simulink model "stateflow_test"  (R2020a)
settings: Solver=FixedStepDiscrete  StartTime=0.0  StopTime=inf  FixedStep=0.01  RelTol=1e-3  EnableMultiTasking=on
settings Model: EnablePacing=on  Creator=HannesDittmann  LastModifiedBy=alf
settings SolverCC: AutoInsertRateTranBlk=on
settings DataIOCC: LimitDataPoints=on  ReturnWorkspaceOutputs=off
settings OptimizationCC: LifeSpan=inf
settings DebuggingCC: AllowSymbolicDim=off  SFUnexpectedBacktrackingDiag=warning  SFNoUnconditionalDefaultTransitionDiag=warning  SFExecutionAtInitializationDiag=none  ArithmeticOperatorsInVariantConditions=warning
settings SFSimCC: SimUseLocalCustomCode=off  CustomCodeUndefinedFunction=UseInterfaceOnly
settings RTWCC: RTWUseLocalCustomCode=off
settings CodeAppCC: StateflowObjectComments=on
settings GRTTargetCC: TargetLangStandard=C89/C90 (ANSI)
settings ConfigComp: CovMetricSettings=dw  CovHtmlReporting=on  CovSaveCumulativeToWorkspaceVar=on  CovSaveSingleToWorkspaceVar=on  CovShowResultsExplorer=off  CovExternalEMLEnable=off

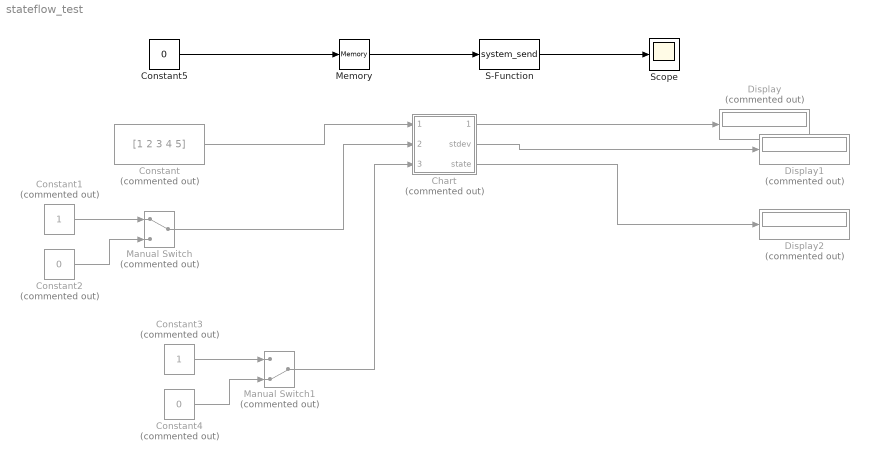
== system stateflow_test ==
  Chart : Stateflow chart  Commented=on  TreatAsAtomicUnit=on
  Constant : Constant  Commented=on  Value=[1 2 3 4 5]
  Constant1 : Constant  Commented=on
  Constant2 : Constant  Commented=on  Value=0
  Constant3 : Constant  Commented=on
  Constant4 : Constant  Commented=on  Value=0
  Constant5 : Constant  Value=0
  Display : Display  Commented=on
  Display1 : Display  Commented=on
  Display2 : Display  Commented=on
  Manual Switch : ManualSwitch  Commented=on
  Manual Switch1 : ManualSwitch  Commented=on  CurrentSetting=0
  Memory : Memory  InitialCondition=1
  S-Function : S-Function  FunctionName=system_send  SFunctionDeploymentMode=off  EnableBusSupport=off
  Scope : Scope
  wires:
  Chart/1(mean) -> Display/1
  Constant/1 -> Chart/1(invals)
  Chart/2(stdev) -> Display1/1
  Manual Switch/1 -> Chart/2(manual)
  Constant1/1 -> Manual Switch/1
  Constant2/1 -> Manual Switch/2
  Constant3/1 -> Manual Switch1/1
  Constant4/1 -> Manual Switch1/2
  Manual Switch1/1 -> Chart/3(manual2)
  Chart/3(state) -> Display2/1
  S-Function/1 -> Scope/1
  Constant5/1 -> Memory/1
  Memory/1 -> S-Function/1

== stateflow chart stateflow_test/Chart ==
  state OFF
    state=0;
  state ON
  state a
    (default) -> (junction 82) : {
        | mean = meanstats(invals);
        | stdev = stdevstats(invals);
        | }
  state a1
  (default) -> OFF
  OFF -> ON : [manual==1]/{state=1}
  ON -> OFF [order 1] : [manual==0]/{state=0}
  ON -> a [order 2] : [(manual2==1)&&(state==1)]/{state=2}
  a1 -> OFF [order 1] : [manual==0 && manual2==0 &&state==3]/{state=0}
  a -> a1 : [manual2==0 && state==2]/{state=3}
  a1 -> a [order 2] : [manual2==1&&state==3]/{state=2}
  data: vals function_input size=5; meanout function_output; vals function_input size=5; stdevout function_output; mean output size=1; stdev output size=1; invals input size=5; manual input; manual2 input; state output
  function meanout  = meanstats(vals):
    | function meanout  = meanstats(vals)
    | %#codegen
    | 
    | % Calculates the statistical mean for vals
    | 
    | len = length(vals);
    | meanout = avg(vals,len);
    | 
    | coder.extrinsic('plot');
    | plot(vals,'-+');
    | 
    | system('mkdir neu');
    | 
    | function mean = avg(array,size)
    | mean = sum(array)/size;
  function stdevout = stdevstats(vals):
    | function stdevout = stdevstats(vals)
    | %#codegen
    | 
    | % Calculates the standard deviation for vals
    | 
    | len = length(vals);
    | stdevout = sqrt(sum(((vals-avg(vals,len)).^2))/len);
    | 
    | function mean = avg(array,size)
    | mean = sum(array)/size;
